simulink model "MagnetoShield_PID_Nonlinear_Simulation_CT"  (R2019a)
settings: Solver=VariableStepAuto  StartTime=0.0  StopTime=15  RelTol=1e-3
undefined symbols (not defined in the file): C, g, Ke, Km, L, m, R, sigbuilder_block
libraries: simulink x1
settings Model: Creator=jakub  LastModifiedBy=jakub

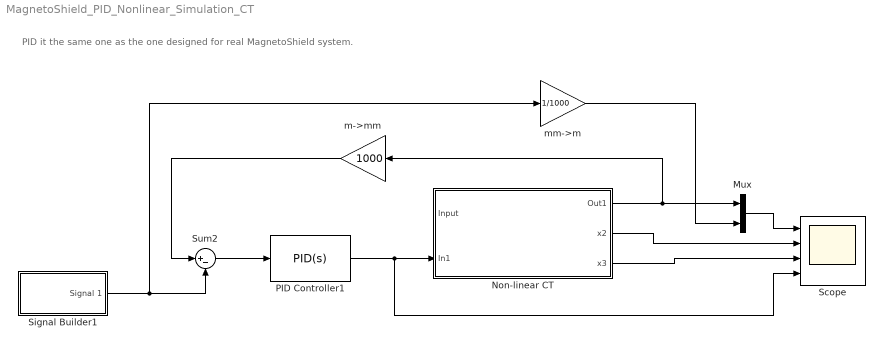
== system MagnetoShield_PID_Nonlinear_Simulation_CT ==
  note: PID it the same one as the one designed for real MagnetoShield system.
  Mux : Mux  Inputs=2
  Non-linear CT : Subsystem
  PID Controller1 : simulink/Continuous/PID Controller  Controller=PID  Form=Parallel  TimeDomain=Continuous-time  SampleTime=-1  IntegratorMethod=Forward Euler  FilterMethod=Forward Euler  ControllerParametersSource=internal  P=3.5  I=1/0.6  D=0.025  UseFilter=on  N=100  TunerSelectOption=Transfer Function Based (PID Tuner App)  InitialConditionSource=internal  InitialConditionForIntegrator=0  InitialConditionForFilter=0  DifferentiatorICPrevScaledInput=0  ExternalReset=none  TrackingMode=off  Kt=1  LimitOutput=on  UpperSaturationLimit=10  LowerSaturationLimit=0  LinearizeAsGain=on  AntiWindupMode=none  Kb=1  POutMin=[]  POutMax=[]  IOutMin=[]  IOutMax=[]  DOutMin=[]  DOutMax=[]  NOutMin=[]  NOutMax=[]  SumOutMin=[]  SumOutMax=[]  SaturationOutMin=[]  SaturationOutMax=[]  PParamMin=[]  PParamMax=[]  IParamMin=[]  IParamMax=[]  DParamMin=[]  DParamMax=[]  NParamMin=[]  NParamMax=[]  KbParamMin=[]  KbParamMax=[]  KtParamMin=[]  KtParamMax=[]  KbOutMin=[]  KbOutMax=[]  KtOutMin=[]  KtOutMax=[]  IntegratorOutMin=[]  IntegratorOutMax=[]  FilterOutMin=[]  FilterOutMax=[]  SumI1OutMin=[]  SumI1OutMax=[]  SumI2OutMin=[]  SumI2OutMax=[]  SumI3OutMin=[]  SumI3OutMax=[]  SumI4OutMin=[]  SumI4OutMax=[]  SumDOutMin=[]  SumDOutMax=[]  DifferentiatorOutMin=[]  DifferentiatorOutMax=[]  FilterDiffOutCoefMin=[]  FilterDiffOutCoefMax=[]  ReciprocalOutMin=[]  ReciprocalOutMax=[]  SumDenOutMin=[]  SumDenOutMax=[]  SumNumOutMin=[]  SumNumOutMax=[]  DivideOutMin=[]  DivideOutMax=[]  IntegratorContinuousStateAttributes=''  IntegratorStateMustResolveToSignalObject=off  IntegratorRTWStateStorageClass=Auto  FilterContinuousStateAttributes=''  FilterStateMustResolveToSignalObject=off  FilterRTWStateStorageClass=Auto  ParallelPVariant=InternalParameters  IdealPVariant=Disabled  IVariant=InternalParameters  DVariant=InternalParameters  IntegratorVariant=Continuous  SatVariant=Enabled  AWVariant=Passthrough  PCopyVariant=Disabled  TRVariant=Disabled  FdbkBlocksVariant=Forward  IdealPFdbkVariant=Disabled  SatFdbkVariant=Disabled  DerivativeFilterVariant=ContFilter  NVariant=InternalParameters  NCopyVariant=Disabled  FilterICVariant=InternalICsFilter  IntegratorICVariant=InternalICs  ExternalResetVariant=Disabled  TRSumVariant=Passthrough  SumFdbkVariant=Disabled  SumVariant=Sum_PID
  Scope : Scope  NumInputPorts=4
  Signal Builder1 : Subsystem  Tag=STV Subsys  LoadFcn=sigbuilder_block('load');  StartFcn=sigbuilder_block('start');  StopFcn=sigbuilder_block('stop');  ClipboardFcn=sigbuilder_block('clipboard');  mask(Sigbuilder block){tuvar=[0:10]}
      mask help: Simulink:masks:SigbuilderBlock_MD
      mask init:
      | if ~strcmp(get_param(bdroot(gcbh),'SimulationStatus'),'stopped') tuvar = sigbuilder_block('maskInit'); end
      settings: CopyFcn=sigbuilder_block('copy');  DeleteFcn=sigbuilder_block('delete');  ModelCloseFcn=sigbuilder_block('modelClose');  PreSaveFcn=sigbuilder_block('preSave');  PauseFcn=sigbuilder_block('pause');  ContinueFcn=sigbuilder_block('continue');  NameChangeFcn=sigbuilder_block('namechange');  OpenFcn=sigbuilder_block('open',[434.4 169.8 550.8 400.2 ]);  CloseFcn=sigbuilder_block('close');
      mask Display: plot(0, 0, 100, 100,[2, 2, 32, 32, 2], [68, 8, 8, 68, 68],[32, 2], [38, 38], [32, 19, 2],[53, 60, 44], [32, 17, 17, 2],[16, 16, 31, 31]);txt = getActiveGroup(gcbh);text(2, 100, txt,'verticalAlignment', 'top');
  Sum2 : Sum  Inputs=|+-
  m->mm : Gain  Gain=1000
  mm->m : Gain  Gain=1/1000
  wires:
  Sum2/1 -> PID Controller1/1
  Signal Builder1/1(Signal 1) -> mm->m/1, Sum2/2
  PID Controller1/1 -> Non-linear CT/2(In1), Scope/4
  m->mm/1 -> Sum2/1
  Non-linear CT/2(x2) -> Scope/2
  Non-linear CT/3(x3) -> Scope/3
  Non-linear CT/1(Out1) -> Mux/1, m->mm/1
  mm->m/1 -> Mux/2
  Mux/1 -> Scope/1

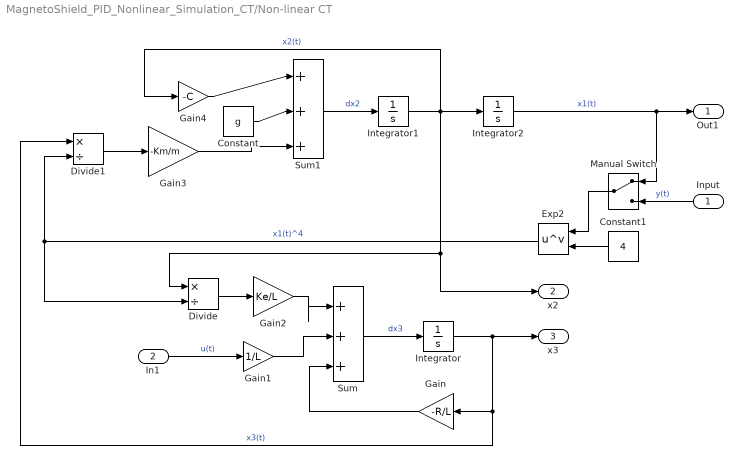
== system MagnetoShield_PID_Nonlinear_Simulation_CT/Non-linear CT ==
  Input : Inport
  In1 : Inport  Port=2
  Constant : Constant  Value=g
  Constant1 : Constant  Value=4
  Divide : Product  Inputs=*/
  Divide1 : Product  Inputs=*/
  Exp2 : Math  Operator=pow  SaturateOnIntegerOverflow=on
  Gain : Gain  Gain=-R/L
  Gain1 : Gain  Gain=1/L
  Gain2 : Gain  Gain=Ke/L
  Gain3 : Gain  Gain=-Km/m
  Gain4 : Gain  Gain=-C
  Integrator : Integrator
  Integrator1 : Integrator
  Integrator2 : Integrator  InitialCondition=0.017
  Manual Switch : ManualSwitch
  Sum : Sum  Inputs=|+++
  Sum1 : Sum  Inputs=|+++
  Out1 : Outport
  x2 : Outport  Port=2
  x3 : Outport  Port=3
  wires:
  Integrator2/1 -> Out1/1, Manual Switch/1  "x1(t)"
  Integrator1/1 -> Gain4/1, x2/1, Divide/1, Integrator2/1  "x2(t)"
  Divide1/1 -> Gain3/1
  Integrator/1 -> x3/1, Gain/1, Divide1/1  "x3(t)"
  Sum1/1 -> Integrator1/1  "dx2"
  Gain2/1 -> Sum/1
  Gain/1 -> Sum/3
  Gain4/1 -> Sum1/1
  Exp2/1 -> Divide1/2, Divide/2  "x1(t)^4"
  Sum/1 -> Integrator/1  "dx3"
  Constant1/1 -> Exp2/2
  Gain3/1 -> Sum1/3
  Constant/1 -> Sum1/2
  In1/1 -> Gain1/1  "u(t)"
  Gain1/1 -> Sum/2
  Divide/1 -> Gain2/1
  Manual Switch/1 -> Exp2/1
  Input/1 -> Manual Switch/2  "y(t)"

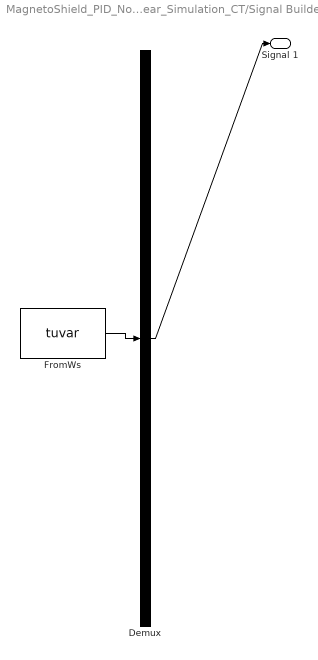
== system MagnetoShield_PID_Nonlinear_Simulation_CT/Signal Builder1 ==
  Demux : Demux  Tag=STV Demux  Outputs=1
  FromWs : FromWorkspace  Tag=STV FromWs  VariableName=tuvar  SampleTime=0
      SigBuilderData=|
      | common.afterFinalStr = 'Extrapolate'
      | common.sampleTime = 0
      | dataSet.timeRange = [0 15]
      | dataSet.name = 'Group 1'
      | sbobj.Groups.Name = 'Group 1'
      | sbobj.Groups.Signals.Name = 'Signal 1'
      | sbobj.Groups.Signals.XData = [0 2 2 4 4 6 6 8 10 12 14 14 15]
      | sbobj.Groups.Signals.YData = [15.5 15.5 14 14 12.5 12.5 14.5 14.5 17 12 14.5 15 15]
      | sbobj.Groups.TimeRange = [0 15]
  Signal 1 : Outport  Tag=STV Outport
  wires:
  FromWs/1 -> Demux/1
  Demux/1 -> Signal 1/1
